simulink model "AdaptivePID_2014a"  (R2014a)
settings: Solver=ode3  SolverMode=SingleTasking  StartTime=0.0  StopTime=10  FixedStep=0.001  RelTol=1e-3
values from neighbouring files (symbols this model uses):
  F1 = 2*wc    (= 80)    [Para.m]
  F2 = wc^2    (= 1600)    [Para.m]
  k00 = 0    [Para.m]
  k10 = 0    [Para.m]
  k20 = 0    [Para.m]
  namuta0 = 1000    [Para.m]
  namuta1 = 1000    [Para.m]
  namuta2 = 1000    [Para.m]
  p1 = 10    [Para.m]
  p2 = 1    [Para.m]
settings Model: CovMetricSettings=dwe  CovHtmlReporting=off  covSaveCumulativeToWorkspaceVar=off  CovSaveSingleToWorkspaceVar=off  CovExternalEMLEnable=on  CovSFcnEnable=on  Creator=chengqian  LastModifiedBy=chengqian
settings DataIOCC: LimitDataPoints=off  SaveFormat=StructureWithTime
settings DebuggingCC: MergeDetectMultiDrivingBlocksExec=error  SolverPrmCheckMsg=none  FrameProcessingCompatibilityMsg=error  SFUnexpectedBacktrackingDiag=error  SFNoUnconditionalDefaultTransitionDiag=error
settings HardwareCC: ProdBitPerPointer=64  ProdLargestAtomicFloat=Float  ProdIntDivRoundTo=Zero  ProdEndianess=LittleEndian  ProdHWDeviceType=Specified
settings ModelReferenceCC: PropagateSignalLabelsOutOfModel=on
settings SFSimCC: SimUseLocalCustomCode=on
settings RTWCC: RTWUseLocalCustomCode=on
settings GRTTargetCC: TargetLangStandard=C99 (ISO)  GeneratePreprocessorConditionals=Use local settings

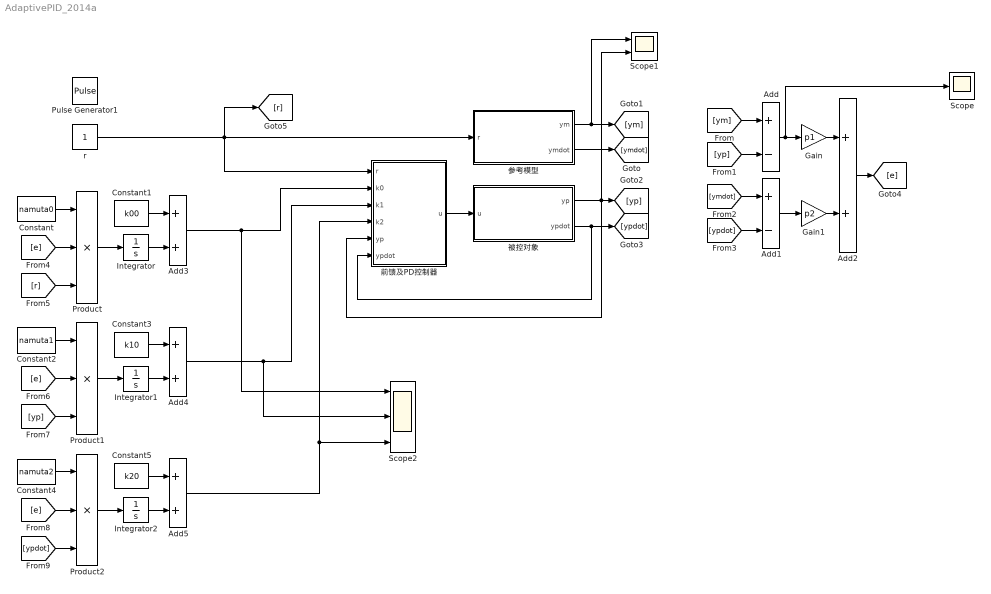
== system AdaptivePID_2014a ==
  Add : Sum  Inputs=+-
  Add1 : Sum  Inputs=+-
  Add{2..5} (4 alike) : Sum
  Constant : Constant  Value=namuta0
  Constant1 : Constant  Value=k00
  Constant2 : Constant  Value=namuta1
  Constant3 : Constant  Value=k10
  Constant4 : Constant  Value=namuta2
  Constant5 : Constant  Value=k20
  Gain : Gain  Gain=p1
  Gain1 : Gain  Gain=p2
  Integrator : Integrator
  Integrator1 : Integrator
  Integrator2 : Integrator
  Product : Product  Inputs=3
  Product1 : Product  Inputs=3
  Product2 : Product  Inputs=3
  Pulse Generator1 : DiscretePulseGenerator  PulseType=Time based  PulseWidth=50
  Scope : Scope
      settings: TimeRange=auto  MaxDataPoints=5000  SaveToWorkspace=off  SaveName=ScopeData  YMin=-0.07986  YMax=0.24352  SampleTime=-1
  Scope1 : Scope  NumInputPorts=2
      settings: TimeRange=auto  MaxDataPoints=5000  SaveToWorkspace=off  YMin=-0.13094~-5  YMax=1.17844~5  SampleTime=-1
  Scope2 : Scope  NumInputPorts=3
      settings: TimeRange=auto  MaxDataPoints=5000  SaveToWorkspace=off  SaveName=ScopeData2  YMin=-360.9463~-5~-5  YMax=366.90037~5~5  SampleTime=-1
  r : Constant
  前馈及PD控制器 : MATLAB Function  TreatAsAtomicUnit=on
      settings: PermitHierarchicalResolution=ParametersOnly
  参考模型 : Subsystem
  被控对象 : Subsystem
  wires:
  前馈及PD控制器/1(u) -> 被控对象/1(u)
  参考模型/2(ymdot) -> [ymdot]
  参考模型/1(ym) -> Scope1/1, [ym]
  被控对象/2(ypdot) -> 前馈及PD控制器/6(ypdot), [ypdot]
  被控对象/1(yp) -> Scope1/2, 前馈及PD控制器/5(yp), [yp]
  [ym] -> Add/1
  [yp] -> Add/2
  Add/1 -> Scope/1, Gain/1
  [ymdot] -> Add1/1
  [ypdot] -> Add1/2
  Add1/1 -> Gain1/1
  Gain/1 -> Add2/1
  Gain1/1 -> Add2/2
  Add2/1 -> [e]
  Constant/1 -> Product/1
  [e] -> Product/2
  [r] -> Product/3
  Product/1 -> Integrator/1
  Integrator/1 -> Add3/2
  Constant1/1 -> Add3/1
  Integrator1/1 -> Add4/2
  Constant2/1 -> Product1/1
  Constant3/1 -> Add4/1
  Product1/1 -> Integrator1/1
  [e] -> Product1/2
  [yp] -> Product1/3
  Integrator2/1 -> Add5/2
  Constant4/1 -> Product2/1
  Constant5/1 -> Add5/1
  Product2/1 -> Integrator2/1
  [e] -> Product2/2
  [ypdot] -> Product2/3
  Add3/1 -> Scope2/1, 前馈及PD控制器/2(k0)
  Add4/1 -> Scope2/2, 前馈及PD控制器/3(k1)
  Add5/1 -> Scope2/3, 前馈及PD控制器/4(k2)
  r/1 -> [r], 参考模型/1(r), 前馈及PD控制器/1(r)

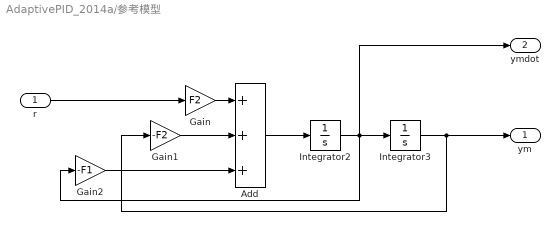
== system AdaptivePID_2014a/参考模型 ==
  r : Inport
  Add : Sum  Inputs=+++
  Gain : Gain  Gain=F2
  Gain1 : Gain  Gain=-F2
  Gain2 : Gain  Gain=-F1
  Integrator2 : Integrator
  Integrator3 : Integrator
  ym : Outport
  ymdot : Outport  Port=2
  wires:
  Gain2/1 -> Add/3
  r/1 -> Gain/1
  Integrator2/1 -> Gain2/1, ymdot/1, Integrator3/1
  Integrator3/1 -> ym/1, Gain1/1
  Add/1 -> Integrator2/1
  Gain/1 -> Add/1
  Gain1/1 -> Add/2

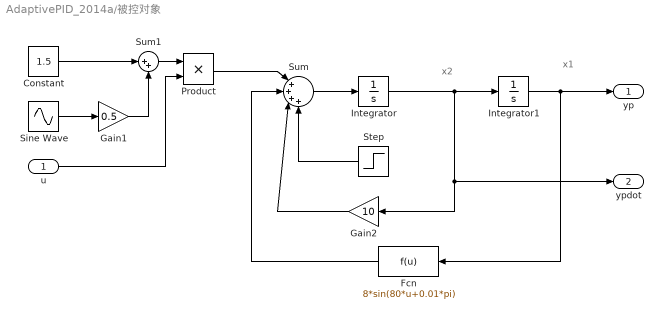
== system AdaptivePID_2014a/被控对象 ==
  note: x2
  note: x1
  u : Inport
  Constant : Constant  Value=1.5
  Fcn : Fcn  Expr=8*sin(80*u+0.01*pi)
  Gain1 : Gain  Gain=0.5
  Gain2 : Gain  Gain=10
  Integrator : Integrator
  Integrator1 : Integrator
  Product : Product
  Sine Wave : Sin  Bias=1  Frequency=0.2*pi  SampleTime=0
  Step : Step  Time=5  After=100  SampleTime=0
  Sum : Sum  Inputs=|++++
  Sum1 : Sum  Inputs=|++
  yp : Outport
  ypdot : Outport  Port=2
  wires:
  Fcn/1 -> Sum/2
  Gain2/1 -> Sum/3
  Product/1 -> Sum/1
  Sine Wave/1 -> Gain1/1
  Sum1/1 -> Product/1
  Gain1/1 -> Sum1/2
  Integrator/1 -> Integrator1/1, ypdot/1, Gain2/1
  Constant/1 -> Sum1/1
  u/1 -> Product/2
  Integrator1/1 -> yp/1, Fcn/1
  Sum/1 -> Integrator/1
  Step/1 -> Sum/4

== matlab function AdaptivePID_2014a/前馈及PD控制器 ==
  data: r input; k0 input; k1 input; k2 input; u output; yp input; ypdot input
function u = fcn(r,k0,k1,k2,yp,ypdot)

u = r*k0 + yp*k1 + ypdot*k2;
